simulink model "sampleModel2015"  (R2023a)
settings: Solver=VariableStepAuto  StartTime=0.0  StopTime=10.0  RelTol=1e-3
libraries: simulink x7, hdlsllib x7
settings Model: Creator=user1  LastModifiedBy=user1

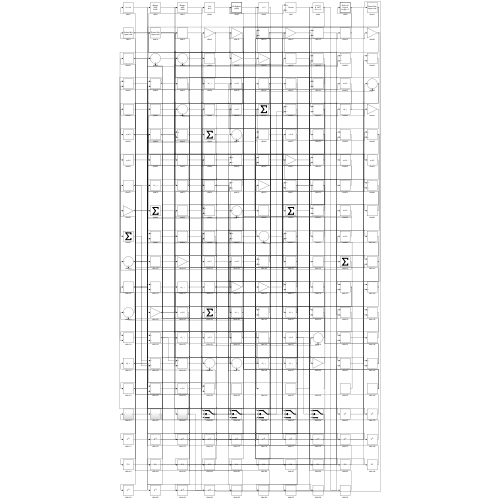
[thumbnail: Simulink's stored preview of the top-level diagram]
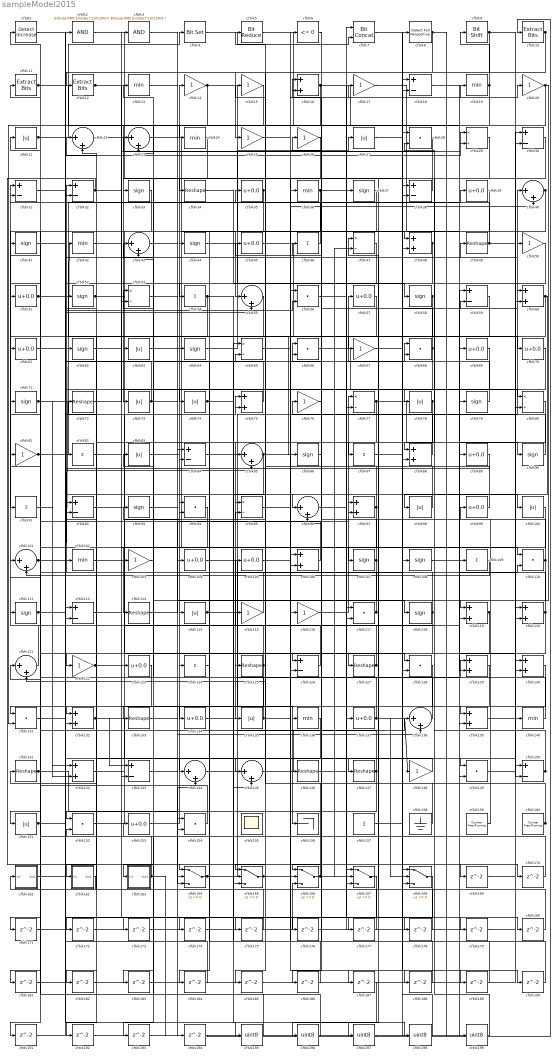
== system sampleModel2015 ==
  cfblk1 : simulink/Logic and Bit Operations/Detect Increase  vinit=0.0  OutDataTypeStr=boolean
      settings: LibrarySourceBlock=|
      | hdlsllib/Logic and Bit
      | Operations/Detect
      | Increase
  cfblk10 : simulink/Logic and Bit Operations/Extract Bits  bitsToExtract=Upper half  numBits=8  bitIdxRange=[0 7]  outScalingMode=Preserve fixed-point scaling
      settings: LibrarySourceBlock=|
      | hdlsllib/Logic and Bit
      | Operations/Extract Bits
  cfblk{21,27,63,73..74,78,83,98,100,114,135,151} (12 alike) : Abs  SaturateOnIntegerOverflow=off
  cfblk{22..23,40,43,55,85,96,101,121,138,144..145} (12 alike) : Sum  Inputs=|++
  cfblk{13,19,24,36,42,102,136,140} (8 alike) : MinMax
  cfblk{14..15,17,20,25..26,50,67,76,81,103,115..116,122,148} (15 alike) : Gain
  cfblk{35,39,45,51,57,61,69..70,89,99,104..105,123,134,137,153} (16 alike) : Bias  Bias=0.0  SaturateOnIntegerOverflow=off
  cfblk{16,48,60,75,88,97,106,119..120,129..130,132,139,142} (14 alike) : Sum
  cfblk{33,37,41,44,52,58,62,64,71,79,86,90,93,107..108,111,118} (17 alike) : Signum
  cfblk{46,54,82,87,91,109,124} (7 alike) : Sum  Inputs=+
  cfblk11 : simulink/Logic and Bit Operations/Extract Bits  bitsToExtract=Upper half  numBits=8  bitIdxRange=[0 7]  outScalingMode=Preserve fixed-point scaling
      settings: LibrarySourceBlock=|
      | hdlsllib/Logic and Bit
      | Operations/Extract Bits
  cfblk{28,56,66,68,94,110,117,128,131,149,152,154} (12 alike) : DotProduct  OutDataTypeStr=Inherit: Inherit via internal rule
  cfblk{18,30..32,38,59,84,92,112,126,143,150} (12 alike) : Sum  Inputs=+-
  cfblk{34,49,72,113,125,127,133,141,146..147} (10 alike) : Reshape
  cfblk12 : simulink/Logic and Bit Operations/Extract Bits  bitsToExtract=Upper half  numBits=8  bitIdxRange=[0 7]  outScalingMode=Preserve fixed-point scaling
      settings: LibrarySourceBlock=|
      | hdlsllib/Logic and Bit
      | Operations/Extract Bits
  cfblk155 : Scope
      settings: Floating=on
  cfblk156 : Terminator
  cfblk157 : Constant  SampleTime=-1
  cfblk158 : Ground
  cfblk159 : hdlsllib/Sources/Counter Free-Running  NumBits=16  tsamp=-1
  cfblk160 : hdlsllib/Sources/Counter Free-Running  NumBits=16  tsamp=-1
  cfblk161 : Subsystem
      settings: LibrarySourceBlock=|
      | hdlsllib/Ports &
      | Subsystems/Subsystem
  cfblk162 : Subsystem
      settings: LibrarySourceBlock=|
      | hdlsllib/Ports &
      | Subsystems/Subsystem
  cfblk163 : Subsystem
      settings: LibrarySourceBlock=|
      | hdlsllib/Ports &
      | Subsystems/Subsystem
  cfblk{164..168} (5 alike) : Switch  SaturateOnIntegerOverflow=off  InputSameDT=off
  cfblk{169..194} (26 alike) : Delay  SampleTime=1
  cfblk{195..199} (5 alike) : DataTypeConversion  OutDataTypeStr=uint8  SaturateOnIntegerOverflow=off  RndMeth=Floor
  cfblk2 : simulink/Logic and Bit Operations/Bitwise Operator  logicop=AND  UseBitMask=on  BitMask=bin2dec('11011001')  BitMaskRealWorld=Stored Integer
      settings: LibrarySourceBlock=|
      | hdlsllib/Logic and Bit
      | Operations/Bitwise
      | Operator
  cfblk{29,47,53,65,77,80,95} (7 alike) : Product  Inputs=*/  RndMeth=Zero  SaturateOnIntegerOverflow=on
  cfblk3 : simulink/Logic and Bit Operations/Bitwise Operator  logicop=AND  UseBitMask=on  BitMask=bin2dec('11011001')  BitMaskRealWorld=Stored Integer
      settings: LibrarySourceBlock=|
      | hdlsllib/Logic and Bit
      | Operations/Bitwise
      | Operator
  cfblk4 : simulink/Logic and Bit Operations/Bit Set  iBit=0
      settings: LibrarySourceBlock=|
      | hdlsllib/Logic and Bit
      | Operations/Bit Set
  cfblk5 : hdlsllib/Logic and Bit Operations/Bit Reduce  mode=AND
  cfblk6 : hdlsllib/Logic and Bit Operations/Compare To Zero  relop=<=  OutDataTypeStr=boolean
  cfblk7 : hdlsllib/Logic and Bit Operations/Bit Concat  numInputs=2
  cfblk8 : hdlsllib/Logic and Bit Operations/Detect Fall Nonpositive  vinit=0  OutDataTypeStr=boolean
  cfblk9 : hdlsllib/Logic and Bit Operations/Bit Shift  mode=Shift Left Logical  N=0
  wires:
  cfblk64/1 -> cfblk27/1
  cfblk90/1 -> cfblk76/1
  cfblk60/1 -> cfblk98/1, cfblk168/3
  cfblk24/1 -> cfblk110/1
  cfblk58/1 -> cfblk86/1, cfblk85/1
  cfblk33/1 -> cfblk127/1
  cfblk91/1 -> cfblk142/1
  cfblk81/1 -> cfblk39/1, cfblk85/2
  cfblk83/1 -> cfblk14/1
  cfblk115/1 -> cfblk32/1
  cfblk20/1 -> cfblk119/1, cfblk23/2
  cfblk61/1 -> cfblk49/1
  cfblk92/1 -> cfblk75/1
  cfblk119/1 -> cfblk141/1, cfblk122/1
  cfblk153/1 -> cfblk44/1
  cfblk123/1 -> cfblk132/1
  cfblk160/1 -> cfblk93/1, cfblk47/1, cfblk121/2
  cfblk14/1 -> cfblk48/1, cfblk131/2
  cfblk99/1 -> cfblk31/1
  cfblk4/1 -> cfblk7/2
  cfblk150/1 -> cfblk114/1, cfblk23/1
  cfblk152/1 -> cfblk94/1
  cfblk88/1 -> cfblk66/1
  cfblk48/1 -> cfblk166/1, cfblk167/2
  cfblk130/1 -> cfblk139/1
  cfblk134/1 -> cfblk40/1
  cfblk94/1 -> cfblk113/1
  cfblk22/1 -> cfblk73/1
  cfblk116/1 -> cfblk77/1
  cfblk46/1 -> cfblk35/1
  cfblk21/1 -> cfblk4/1, cfblk143/2
  cfblk164/1 -> cfblk129/1, cfblk59/2
  cfblk166/1 -> cfblk37/1, cfblk47/2, cfblk95/2
  cfblk65/1 -> cfblk20/1
  cfblk34/1 -> cfblk58/1
  cfblk112/1 -> cfblk149/1
  cfblk32/1 -> cfblk164/1, cfblk178/1
  cfblk35/1 -> cfblk151/1, cfblk74/1, cfblk175/1
  cfblk17/1 -> cfblk69/1
  cfblk26/1 -> cfblk63/1
  cfblk84/1 -> cfblk135/1
  cfblk133/1 -> cfblk164/2
  cfblk120/1 -> cfblk147/1, cfblk43/2
  cfblk104/1 -> cfblk156/1
  cfblk121/1 -> cfblk31/2
  cfblk79/1 -> cfblk57/1
  cfblk101/1 -> cfblk42/1, cfblk56/2, cfblk29/2
  cfblk36/1 -> cfblk128/1, cfblk51/1
  cfblk63/1 -> cfblk168/1
  cfblk148/1 -> cfblk144/1
  cfblk149/1 -> cfblk30/2
  cfblk57/1 -> cfblk91/1
  cfblk16/1 -> cfblk79/1, cfblk53/2, cfblk179/1
  cfblk59/1 -> cfblk134/1
  cfblk15/1 -> cfblk33/1
  cfblk147/1 -> cfblk152/1, cfblk81/1
  cfblk163/1(Out1) -> cfblk11/1, cfblk194/1
  cfblk68/1 -> cfblk164/3, cfblk16/1
  cfblk74/1 -> cfblk126/2, cfblk198/1
  cfblk76/1 -> cfblk26/1
  cfblk11/1 -> cfblk104/1, cfblk88/2
  cfblk139/1 -> cfblk120/1
  cfblk107/1 -> cfblk163/1(In1), cfblk45/1
  cfblk67/1 -> cfblk8/1
  cfblk56/1 -> cfblk137/1
  cfblk50/1 -> cfblk54/1
  cfblk137/1 -> cfblk148/1, cfblk168/2, cfblk41/1
  cfblk40/1 -> cfblk176/1, cfblk177/1
  cfblk122/1 -> cfblk38/1, cfblk52/1, cfblk165/2
  cfblk113/1 -> cfblk97/1
  cfblk118/1 -> cfblk83/1, cfblk191/1
  cfblk37/1 -> cfblk61/1
  cfblk159/1 -> cfblk99/1
  cfblk110/1 -> cfblk82/1, cfblk184/1
  cfblk77/1 -> cfblk90/1, cfblk60/1, cfblk87/1
  cfblk106/1 -> cfblk21/1
  cfblk140/1 -> cfblk92/1
  cfblk125/1 -> cfblk111/1, cfblk183/1
  cfblk96/1 -> cfblk19/1
  cfblk13/1 -> cfblk80/1
  cfblk142/1 -> cfblk59/1
  cfblk97/1 -> cfblk65/2, cfblk165/1
  cfblk42/1 -> cfblk103/1
  cfblk30/1 -> cfblk88/1
  cfblk49/1 -> cfblk80/2, cfblk15/1
  cfblk162/1(Out1) -> cfblk161/1(In1)
  cfblk85/1 -> cfblk68/1, cfblk165/3
  cfblk69/1 -> cfblk128/2
  cfblk144/1 -> cfblk36/1
  cfblk128/1 -> cfblk162/1(In1)
  cfblk19/1 -> cfblk9/1, cfblk24/1
  cfblk66/1 -> cfblk109/1
  cfblk9/1 -> cfblk140/1, cfblk115/1
  cfblk23/1 -> cfblk55/1
  cfblk127/1 -> cfblk22/2, cfblk126/1, cfblk16/2
  cfblk45/1 -> cfblk150/1
  cfblk25/1 -> cfblk17/1
  cfblk73/1 -> cfblk62/1, cfblk117/2
  cfblk146/1 -> cfblk167/1
  cfblk47/1 -> cfblk92/2
  cfblk3/1 -> cfblk38/2
  cfblk158/1 -> cfblk124/1
  cfblk41/1 -> cfblk96/1
  cfblk10/1 -> cfblk25/1, cfblk12/1
  cfblk70/1 -> cfblk112/2
  cfblk103/1 -> cfblk53/1
  cfblk44/1 -> cfblk106/2
  cfblk132/1 -> cfblk150/2, cfblk143/1
  cfblk75/1 -> cfblk43/1
  cfblk71/1 -> cfblk75/2, cfblk142/2
  cfblk165/1 -> cfblk40/2, cfblk187/1
  cfblk126/1 -> cfblk105/1
  cfblk102/1 -> cfblk123/1
  cfblk161/1(Out1) -> cfblk102/1
  cfblk51/1 -> cfblk116/1, cfblk117/1
  cfblk2/1 -> cfblk84/1
  cfblk145/1 -> cfblk138/1
  cfblk143/1 -> cfblk154/1
  cfblk108/1 -> cfblk110/2
  cfblk12/1 -> cfblk146/1, cfblk145/1, cfblk107/1
  cfblk157/1 -> cfblk108/1
  cfblk138/1 -> cfblk13/1
  cfblk8/1 -> cfblk95/1, cfblk199/1
  cfblk72/1 -> cfblk3/1
  cfblk109/1 -> cfblk101/2
  cfblk100/1 -> cfblk131/1
  cfblk78/1 -> cfblk172/1, cfblk173/1
  cfblk5/1 -> cfblk77/2
  cfblk131/1 -> cfblk2/1
  cfblk151/1 -> cfblk32/2, cfblk68/2
  cfblk7/1 -> cfblk70/1
  cfblk43/1 -> cfblk125/1
  cfblk154/1 -> cfblk121/1
  cfblk29/1 -> cfblk133/1
  cfblk141/1 -> cfblk154/2, cfblk50/1
  cfblk27/1 -> cfblk100/1
  cfblk80/1 -> cfblk129/2
  cfblk111/1 -> cfblk55/2, cfblk167/3, cfblk180/1
  cfblk93/1 -> cfblk138/2
  cfblk117/1 -> cfblk5/1, cfblk71/1
  cfblk89/1 -> cfblk84/2
  cfblk52/1 -> cfblk67/1, cfblk29/1
  cfblk82/1 -> cfblk136/1
  cfblk98/1 -> cfblk46/1
  cfblk62/1 -> cfblk78/1
  cfblk18/1 -> cfblk130/2
  cfblk124/1 -> cfblk64/1
  cfblk38/1 -> cfblk34/1
  cfblk54/1 -> cfblk118/1, cfblk192/1
  cfblk114/1 -> cfblk18/1, cfblk145/2
  cfblk6/1 -> cfblk96/2
  cfblk135/1 -> cfblk6/1, cfblk72/1
  cfblk53/1 -> cfblk169/1
  cfblk169/1 -> cfblk30/1
  cfblk31/1 -> cfblk170/1
  cfblk170/1 -> cfblk101/1
  cfblk129/1 -> cfblk171/1
  cfblk171/1 -> cfblk139/2
  cfblk172/1 -> cfblk56/1
  cfblk173/1 -> cfblk166/3
  cfblk168/1 -> cfblk174/1
  cfblk174/1 -> cfblk7/1
  cfblk175/1 -> cfblk22/1
  cfblk176/1 -> cfblk120/2
  cfblk177/1 -> cfblk152/2
  cfblk178/1 -> cfblk97/2
  cfblk179/1 -> cfblk60/2
  cfblk180/1 -> cfblk166/2
  cfblk55/1 -> cfblk181/1
  cfblk181/1 -> cfblk149/2
  cfblk167/1 -> cfblk182/1
  cfblk182/1 -> cfblk119/2
  cfblk183/1 -> cfblk48/2
  cfblk184/1 -> cfblk112/1
  cfblk136/1 -> cfblk185/1
  cfblk185/1 -> cfblk130/1
  cfblk86/1 -> cfblk186/1
  cfblk186/1 -> cfblk106/1
  cfblk105/1 -> cfblk188/1
  cfblk188/1 -> cfblk66/2
  cfblk87/1 -> cfblk189/1
  cfblk189/1 -> cfblk65/1
  cfblk95/1 -> cfblk190/1
  cfblk190/1 -> cfblk94/2
  cfblk191/1 -> cfblk132/2
  cfblk192/1 -> cfblk18/2
  cfblk39/1 -> cfblk193/1
  cfblk193/1 -> cfblk144/2
  cfblk194/1 -> cfblk10/1
  cfblk1/1 -> cfblk195/1
  cfblk195/1 -> cfblk153/1
  cfblk187/1 -> cfblk196/1
  cfblk196/1 -> cfblk1/1
  cfblk28/1 -> cfblk197/1
  cfblk197/1 -> cfblk89/1
  cfblk198/1 -> cfblk28/1
  cfblk199/1 -> cfblk28/2

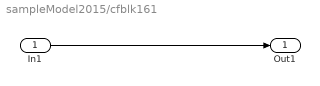
== system sampleModel2015/cfblk161 ==
  In1 : Inport
  Out1 : Outport
  wires:
  In1/1 -> Out1/1

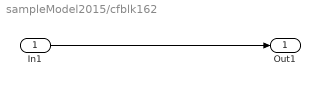
== system sampleModel2015/cfblk162 ==
  In1 : Inport
  Out1 : Outport
  wires:
  In1/1 -> Out1/1

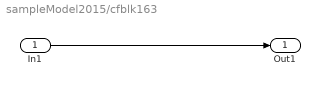
== system sampleModel2015/cfblk163 ==
  In1 : Inport
  Out1 : Outport
  wires:
  In1/1 -> Out1/1
